simulink model "lab5_sim_R2014a"  (R2014a)
settings: Solver=FixedStepDiscrete  SolverMode=SingleTasking  StartTime=1  StopTime=N  FixedStep=1  RelTol=1e-3
values from neighbouring files (symbols this model uses):
  A = [1, 1, 1, 1.3, 1/2]    [lab5.m]
  B = [2, 3, 2, 2, 2]    [lab5.m]
  H = [0,0,0,0,1; 1,0,0,0,0; 0,1,0,0,0; 0,0,1,0,0; 0,0,0,1,0]    [lab5.m]
settings Model: CovMetricSettings=dwe  CovHtmlReporting=off  covSaveCumulativeToWorkspaceVar=off  CovSaveSingleToWorkspaceVar=off  CovExternalEMLEnable=on  CovSFcnEnable=on  Creator=lev  LastModifiedBy=lev
settings DataIOCC: LimitDataPoints=off  SaveFormat=StructureWithTime
settings DebuggingCC: MergeDetectMultiDrivingBlocksExec=error  SolverPrmCheckMsg=none  FrameProcessingCompatibilityMsg=error  SFUnexpectedBacktrackingDiag=error  SFNoUnconditionalDefaultTransitionDiag=error
settings HardwareCC: ProdBitPerPointer=64  ProdLargestAtomicFloat=Float  ProdIntDivRoundTo=Zero  ProdEndianess=LittleEndian  ProdHWDeviceType=Specified
settings ModelReferenceCC: PropagateSignalLabelsOutOfModel=on
settings SFSimCC: SimUseLocalCustomCode=on
settings RTWCC: RTWUseLocalCustomCode=on
settings GRTTargetCC: TargetLangStandard=C99 (ISO)  GeneratePreprocessorConditionals=Use local settings

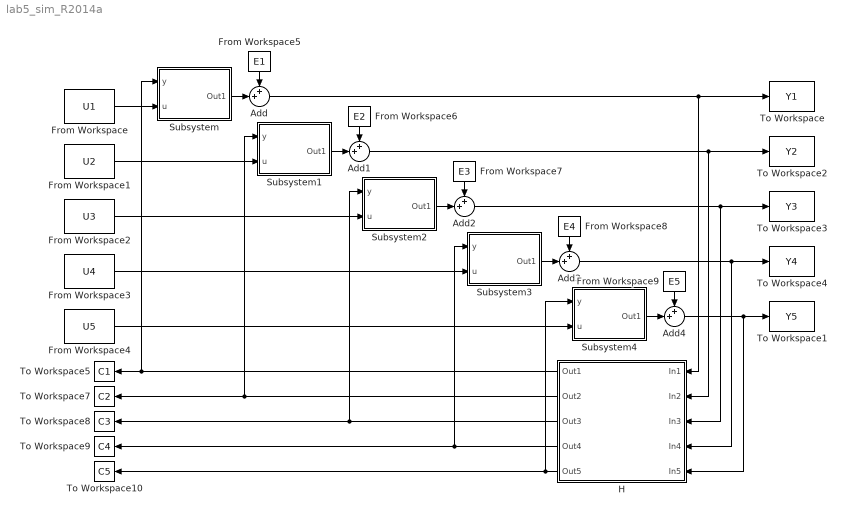
== system lab5_sim_R2014a ==
  Add{,1..4} (5 alike) : Sum  Inputs=++|
  From Workspace : FromWorkspace  VariableName=U1  SampleTime=1  Interpolate=off  OutputAfterFinalValue=Holding final value
  From Workspace1 : FromWorkspace  VariableName=U2  SampleTime=1  Interpolate=off  OutputAfterFinalValue=Holding final value
  From Workspace2 : FromWorkspace  VariableName=U3  SampleTime=1  Interpolate=off  OutputAfterFinalValue=Holding final value
  From Workspace3 : FromWorkspace  VariableName=U4  SampleTime=1  Interpolate=off  OutputAfterFinalValue=Holding final value
  From Workspace4 : FromWorkspace  VariableName=U5  SampleTime=1  Interpolate=off  OutputAfterFinalValue=Holding final value
  From Workspace5 : FromWorkspace  VariableName=E1  SampleTime=0
  From Workspace6 : FromWorkspace  VariableName=E2  SampleTime=0
  From Workspace7 : FromWorkspace  VariableName=E3  SampleTime=0
  From Workspace8 : FromWorkspace  VariableName=E4  SampleTime=0
  From Workspace9 : FromWorkspace  VariableName=E5  SampleTime=0
  H : Subsystem
  Subsystem : Subsystem
  Subsystem1 : Subsystem
  Subsystem2 : Subsystem
  Subsystem3 : Subsystem
  Subsystem4 : Subsystem
  To Workspace : ToWorkspace  VariableName=Y1  SaveFormat=Timeseries  SampleTime=1
  To Workspace1 : ToWorkspace  VariableName=Y5  SaveFormat=Timeseries  SampleTime=1
  To Workspace10 : ToWorkspace  VariableName=C5  SaveFormat=Timeseries  SampleTime=1
  To Workspace2 : ToWorkspace  VariableName=Y2  SaveFormat=Timeseries  SampleTime=1
  To Workspace3 : ToWorkspace  VariableName=Y3  SaveFormat=Timeseries  SampleTime=1
  To Workspace4 : ToWorkspace  VariableName=Y4  SaveFormat=Timeseries  SampleTime=1
  To Workspace5 : ToWorkspace  VariableName=C1  SaveFormat=Timeseries  SampleTime=1
  To Workspace7 : ToWorkspace  VariableName=C2  SaveFormat=Timeseries  SampleTime=1
  To Workspace8 : ToWorkspace  VariableName=C3  SaveFormat=Timeseries  SampleTime=1
  To Workspace9 : ToWorkspace  VariableName=C4  SaveFormat=Timeseries  SampleTime=1
  wires:
  Subsystem/1(Out1) -> Add/2
  Add/1 -> H/1(In1), To Workspace/1
  Subsystem1/1(Out1) -> Add1/2
  Add1/1 -> H/2(In2), To Workspace2/1
  Subsystem2/1(Out1) -> Add2/2
  Add2/1 -> H/3(In3), To Workspace3/1
  Subsystem3/1(Out1) -> Add3/2
  Add3/1 -> H/4(In4), To Workspace4/1
  Subsystem4/1(Out1) -> Add4/2
  From Workspace6/1 -> Add1/1
  From Workspace7/1 -> Add2/1
  From Workspace8/1 -> Add3/1
  From Workspace9/1 -> Add4/1
  From Workspace5/1 -> Add/1
  Add4/1 -> H/5(In5), To Workspace1/1
  From Workspace/1 -> Subsystem/2(u)
  H/5(Out5) -> To Workspace10/1, Subsystem4/1(y)
  H/4(Out4) -> To Workspace9/1, Subsystem3/1(y)
  H/3(Out3) -> To Workspace8/1, Subsystem2/1(y)
  H/2(Out2) -> To Workspace7/1, Subsystem1/1(y)
  H/1(Out1) -> Subsystem/1(y), To Workspace5/1
  From Workspace2/1 -> Subsystem2/2(u)
  From Workspace1/1 -> Subsystem1/2(u)
  From Workspace3/1 -> Subsystem3/2(u)
  From Workspace4/1 -> Subsystem4/2(u)

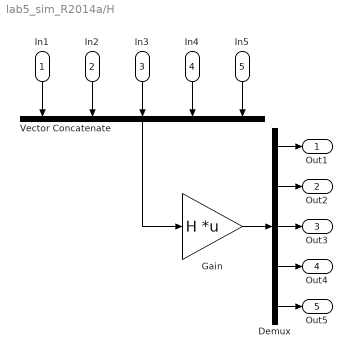
== system lab5_sim_R2014a/H ==
  In1 : Inport
  In2 : Inport  Port=2
  In3 : Inport  Port=3
  In4 : Inport  Port=4
  In5 : Inport  Port=5
  Demux : Demux  Outputs=5
  Gain : Gain  Gain=H  Multiplication=Matrix(K*u) (u vector)  OutDataTypeStr=Inherit: Same as input
  Vector Concatenate : Concatenate  NumInputs=5
  Out1 : Outport
  Out2 : Outport  Port=2
  Out3 : Outport  Port=3
  Out4 : Outport  Port=4
  Out5 : Outport  Port=5
  wires:
  Vector Concatenate/1 -> Gain/1
  Gain/1 -> Demux/1
  Demux/1 -> Out1/1
  Demux/2 -> Out2/1
  Demux/3 -> Out3/1
  Demux/4 -> Out4/1
  Demux/5 -> Out5/1
  In2/1 -> Vector Concatenate/2
  In1/1 -> Vector Concatenate/1
  In4/1 -> Vector Concatenate/4
  In3/1 -> Vector Concatenate/3
  In5/1 -> Vector Concatenate/5

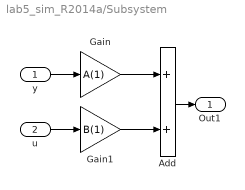
== system lab5_sim_R2014a/Subsystem ==
  y : Inport
  u : Inport  Port=2
  Add : Sum
  Gain : Gain  Gain=A(1)
  Gain1 : Gain  Gain=B(1)
  Out1 : Outport
  wires:
  Add/1 -> Out1/1
  Gain/1 -> Add/1
  Gain1/1 -> Add/2
  y/1 -> Gain/1
  u/1 -> Gain1/1

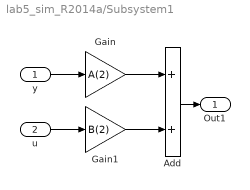
== system lab5_sim_R2014a/Subsystem1 ==
  y : Inport
  u : Inport  Port=2
  Add : Sum
  Gain : Gain  Gain=A(2)
  Gain1 : Gain  Gain=B(2)
  Out1 : Outport
  wires:
  Add/1 -> Out1/1
  Gain/1 -> Add/1
  Gain1/1 -> Add/2
  y/1 -> Gain/1
  u/1 -> Gain1/1

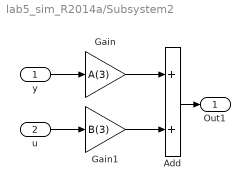
== system lab5_sim_R2014a/Subsystem2 ==
  y : Inport
  u : Inport  Port=2
  Add : Sum
  Gain : Gain  Gain=A(3)
  Gain1 : Gain  Gain=B(3)
  Out1 : Outport
  wires:
  Add/1 -> Out1/1
  Gain/1 -> Add/1
  Gain1/1 -> Add/2
  y/1 -> Gain/1
  u/1 -> Gain1/1

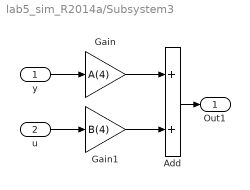
== system lab5_sim_R2014a/Subsystem3 ==
  y : Inport
  u : Inport  Port=2
  Add : Sum
  Gain : Gain  Gain=A(4)
  Gain1 : Gain  Gain=B(4)
  Out1 : Outport
  wires:
  Add/1 -> Out1/1
  Gain/1 -> Add/1
  Gain1/1 -> Add/2
  y/1 -> Gain/1
  u/1 -> Gain1/1

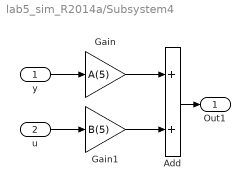
== system lab5_sim_R2014a/Subsystem4 ==
  y : Inport
  u : Inport  Port=2
  Add : Sum
  Gain : Gain  Gain=A(5)
  Gain1 : Gain  Gain=B(5)
  Out1 : Outport
  wires:
  Add/1 -> Out1/1
  Gain/1 -> Add/1
  Gain1/1 -> Add/2
  y/1 -> Gain/1
  u/1 -> Gain1/1
